simulink model "function_block_pump"  (R2023b)
settings: Solver=VariableStepAuto  StartTime=0.0  StopTime=10.0  RelTol=1e-3
libraries: slpidlib x1, nesl_utility x1
settings Model: Creator=pardh  LastModifiedBy=pardh

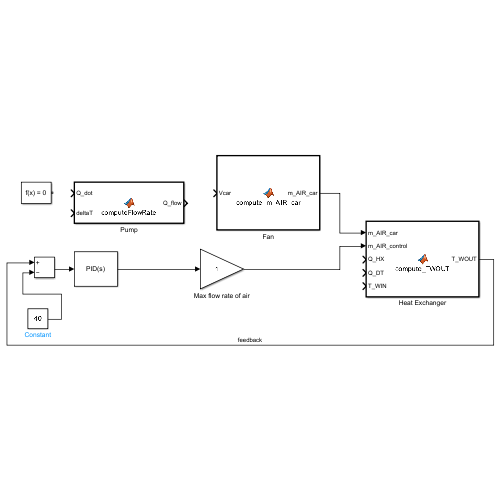
[thumbnail: Simulink's stored preview of the top-level diagram]
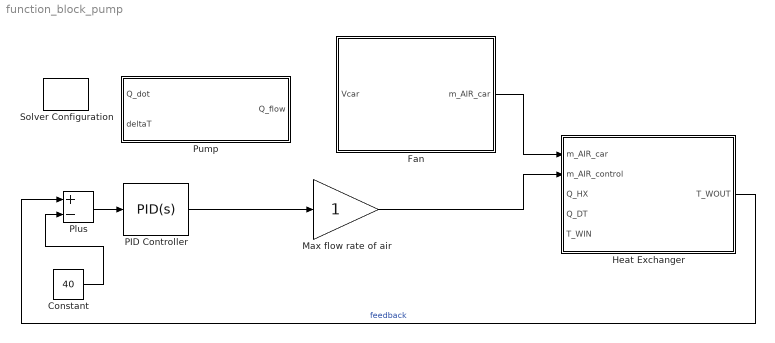
== system function_block_pump ==
  Constant : Constant  Value=40
  Fan : MATLAB Function  TreatAsAtomicUnit=on
  Heat Exchanger : MATLAB Function  TreatAsAtomicUnit=on
  Max flow rate of air : Gain
  PID Controller : slpidlib/PID Controller  Controller=PID  Form=Parallel  TimeDomain=Continuous-time  UseExternalTs=off  SampleTime=-1  IntegratorMethod=Forward Euler  FilterMethod=Forward Euler  ControllerParametersSource=internal  P=1  I=1  UseKiTs=off  D=0  N=100  UseFilter=on  TunerSelectOption=Transfer Function Based (PID Tuner App)  InitialConditionSource=internal  InitialConditionForIntegrator=0  InitialConditionForFilter=0  DifferentiatorICPrevScaledInput=0  ExternalReset=none  TrackingMode=off  Kt=1  LimitOutput=off  SatLimitsSource=internal  UpperSaturationLimit=inf  LowerSaturationLimit=-inf  LinearizeAsGain=on  AntiWindupMode=none  Kb=1  LimitIntegrator=off  UpperIntegratorSaturationLimit=inf  LowerIntegratorSaturationLimit=-inf  POutMin=[]  POutMax=[]  IOutMin=[]  IOutMax=[]  DOutMin=[]  DOutMax=[]  NOutMin=[]  NOutMax=[]  SumOutMin=[]  SumOutMax=[]  SaturationOutMin=[]  SaturationOutMax=[]  PParamMin=[]  PParamMax=[]  IParamMin=[]  IParamMax=[]  DParamMin=[]  DParamMax=[]  NParamMin=[]  NParamMax=[]  KbParamMin=[]  KbParamMax=[]  KtParamMin=[]  KtParamMax=[]  KbOutMin=[]  KbOutMax=[]  KtOutMin=[]  KtOutMax=[]  IntegratorOutMin=[]  IntegratorOutMax=[]  FilterOutMin=[]  FilterOutMax=[]  SumI1OutMin=[]  SumI1OutMax=[]  SumI2OutMin=[]  SumI2OutMax=[]  SumI3OutMin=[]  SumI3OutMax=[]  SumI4OutMin=[]  SumI4OutMax=[]  SumDOutMin=[]  SumDOutMax=[]  DifferentiatorOutMin=[]  DifferentiatorOutMax=[]  FilterDiffOutCoefMin=[]  FilterDiffOutCoefMax=[]  ReciprocalOutMin=[]  ReciprocalOutMax=[]  SumDenOutMin=[]  SumDenOutMax=[]  SumNumOutMin=[]  SumNumOutMax=[]  DivideOutMin=[]  DivideOutMax=[]  UdiffTsProdOutMin=[]  UdiffTsProdOutMax=[]  NTsProdOutMin=[]  NTsProdOutMax=[]  UintegralTsProdOutMin=[]  UintegralTsProdOutMax=[]  UngainTsProdOutMin=[]  UngainTsProdOutMax=[]  ClampingZeroOutDataTypeStr=Inherit: Inherit via back propagation  ClampingZeroOutMin=[]  ClampingZeroOutMax=[]  FilterDenConstantOutDataTypeStr=Inherit: Inherit via back propagation  FilterDenConstantOutMin=[]  FilterDenConstantOutMax=[]  PCopyOutDataTypeStr=Inherit: Inherit via back propagation  PCopyOutMin=[]  PCopyOutMax=[]  NCopyOutDataTypeStr=Inherit: Inherit via back propagation  NCopyOutMin=[]  NCopyOutMax=[]  IntegratorContinuousStateAttributes=''  IntegratorStateMustResolveToSignalObject=off  IntegratorRTWStateStorageClass=Auto  FilterContinuousStateAttributes=''  FilterStateMustResolveToSignalObject=off  FilterRTWStateStorageClass=Auto  ParallelPVariant=InternalParameters  IdealPVariant=Disabled  IVariant=InternalParameters  DVariant=InternalParameters  IntegratorVariant=Continuous  SatVariant=Disabled  AWVariant=Passthrough  PCopyVariant=Disabled  TRVariant=Disabled  FdbkBlocksVariant=Forward  IdealPFdbkVariant=Disabled  SatFdbkVariant=Disabled  DerivativeFilterVariant=ContFilter  NVariant=InternalParameters  NCopyVariant=Disabled  FilterICVariant=InternalICsFilter  IntegratorICVariant=InternalICs  ExternalResetVariant=Disabled  TRSumVariant=Passthrough  SumFdbkVariant=Disabled  SumVariant=Sum_PID  TsampFilterVariant=InternalTs  TsampNgainVariant=Passthrough  TsampIntegralVariant=Passthrough  ExternalSaturationOutDataTypeStr=Inherit: Same as second input
  Plus : Sum  Inputs=+-
  Pump : MATLAB Function  TreatAsAtomicUnit=on
  Solver Configuration : nesl_utility/Solver Configuration  PhysicalDomain=network_engine_domain  SubClassName=solver  LeftPortType=input  RightPortType=generic  Tones=[]  Harmonics=[]  SimulateNoise=off  Profile=off  UseLocalSampling=off  EnableSwitchedLinearOptims=on  FrequencyDomain=off  UseCCode=off  RelTol=0.001  AbsTol=0.001  MinStep=1e-09  ToWorkspace=off  RevertToSquareIcSolve=off  NumHomotopyIterations=100  PhasorMode=off  PhasorModeNumHarmonics=1  ConsistencySolver=NEWTON_XTOL_AFTER_FTOL  IndexReductionMethod=DerivativeReplacement  DoDC=off  ResidualTolerance=1e-09  ConsistencyTolSource=GLOBAL  ConsistencyAbsTol=0.001  ConsistencyRelTol=0.001  ConsistencyTolFactor=0.001  UseLocalSolver=off  LocalSolverChoice=NE_BACKWARD_EULER_ADVANCER  ResolveIndetEquations=on  FunctionEvalNumThread=1  LocalSolverSampleTime=0.001  DoFixedCost=off  MaxNonlinIter=3  MaxModeIter=2  ComputeImpulses=off  ImpulseIterations=2  LinearAlgebra=auto  LinearAlgebraNumThread=0  EquationFormulation=NE_TIME_EF  DelaysMemoryBudget=1024  AutomaticFiltering=on  FilteringTimeConstant=0.001  PartitionStorageMethod=AS_NEEDED  PartitionMemoryBudget=1024  PartitionMethod=ROBUST  MultibodyUseLocalSolver=off  MultibodyLocalSolverChoice=ODE1  MultibodyLocalSolverSampleTime=0.001
  wires:
  PID Controller/1 -> Max flow rate of air/1
  Plus/1 -> PID Controller/1
  Constant/1 -> Plus/2
  Heat Exchanger/1(T_WOUT) -> Plus/1  "feedback"
  Fan/1(m_AIR_car) -> Heat Exchanger/1(m_AIR_car)
  Max flow rate of air/1 -> Heat Exchanger/2(m_AIR_control)

== matlab function function_block_pump/Heat Exchanger ==
  data: m_AIR_car input; m_AIR_control input; T_WOUT output; Q_HX input; Q_DT input; T_WIN input
function T_WOUT = compute_TWOUT(m_AIR_car,m_AIR_control, Q_HX, Q_DT, T_WIN)
% Function to compute T_WOUT using Newton-Raphson method
% Inputs:
% m_AIR - Air mass flow rate (kg/s)
% Q_HX - Heat transfer rate (W)
% Q_DT - Additional heat load (W)
% T_WIN - Water inlet temperature (°C)
% Output:
% T_WOUT - Water outlet temperature (°C)

    % Define constants (modifiable later)
    cp_AIR = 1005; % Specific heat capacity of air (J/kg·K)
    T_AIR_IN = 25; % Air inlet temperature (°C)
    U = 200; % Overall heat transfer coefficient (W/m²·K)
    A = 1.5; % Heat exchanger area (m²)
    F = 1; % Correction factor (unitless)

    % Compute T1
    T1 = T_WIN - (Q_DT / ((m_AIR_control + m_AIR_car) * cp_AIR) + T_AIR_IN);

    % Initial guess for T_WOUT
    T_WOUT = T_AIR_IN + 10; % Reasonable initial guess

    % Tolerance and max iterations
    tol = 1e-6;
    max_iter = 100;
    iter = 0;

    % Newton-Raphson Method
    while iter < max_iter
        T2 = T_WOUT - T_AIR_IN; % T2 = T_WOUT - T_AIR_IN

        % Function to solve (implicit equation)
        f_T2 = T2 - T1 / exp((U * A * F / Q_HX) * (T1 - T2));

        % Derivative (numerical differentiation)
        dT = 1e-6; % Small step for derivative calculation
        f_T2_derivative = ((T2 + dT) - T1 / exp((U * A * F / Q_HX) * (T1 - (T2 + dT))) - f_T2) / dT;

        % Update T2 using Newton-Raphson formula
        T2_new = T2 - f_T2 / f_T2_derivative;

        % Check for convergence
        if abs(T2_new - T2) < tol
            break;
        end

        % Update for next iteration
        T_WOUT = T2_new + T_AIR_IN;
        iter = iter + 1;
    end

    % Ensure output is real (avoid numerical errors)
    T_WOUT = real(T_WOUT);
end

== matlab function function_block_pump/Pump ==
  data: Q_dot input; Q_flow output; deltaT input
function Q_flow = computeFlowRate(Q_dot, deltaT)
% Function to compute required pump flow rate with max limit of 8 LPM

% Constants
Cp = 4200; % Specific heat capacity of water (J/kg·K)
rho = 1000; % Water density (kg/m³)
Q_max = 8; % Maximum flow rate in LPM

% Prevent division by zero
if deltaT < 0.1
    deltaT = 0.1; % Minimum deltaT to avoid infinite flow
end

% Compute mass flow rate (kg/s)
mass_flow_rate = Q_dot / (Cp * deltaT);

% Convert to volumetric flow rate (LPM)
Q_flow = (mass_flow_rate / rho) * 60; 

% Limit flow rate to max 8 LPM
Q_flow = min(Q_flow, Q_max);

end

== matlab function function_block_pump/Fan ==
  data: Vcar input; m_AIR_car output
function m_AIR_car = compute_m_AIR_car(Vcar)
% Compute Q_F based on the given equation (Equation 24)

% Define constants (modify these as per your actual values)
C1 = 5.2; 
C0 = 3.1; 
rho_air = 1.2; 
KR = 0.8; 
A_air1 = 0.5; 
A_air4 = 0.3;

% Compute the denominator term
denominator = (rho_air / 2) * ((KR / (A_air1^2)) + (1 / (A_air4^2)));

% Compute the quadratic equation terms
sqrt_term = sqrt((C1^2) - (4 * denominator * (- (C0 + (rho_air / 2) * (Vcar^2)))));

% Compute Q_F using the quadratic formula (taking the positive root)
m_AIR_car = rho_air *[(-C1 + sqrt_term) / (2 * denominator)];

end
